simulink model "HalfBridgeCapacitanceModeled"  (R2016a)
settings: Solver=FixedStepDiscrete  StartTime=0.0  StopTime=3e-6  FixedStep=SampleTime  RelTol=1e-3
values from neighbouring files (symbols this model uses):
  Dbot = 49    [HalfBridgeCapacitanceModelling.m]
  DelayBot = 50    [HalfBridgeCapacitanceModelling.m]
  DelayTop = 0    [HalfBridgeCapacitanceModelling.m]
  Dtop = 49    [HalfBridgeCapacitanceModelling.m]
  fsw = 1000e3    (= 1000000)    [HalfBridgeCapacitanceModelling.m]
  Rg = 1.5    [HalfBridgeCapacitanceModelling.m]
  Rload = 200/15    (= 13.3333333333)    [HalfBridgeCapacitanceModelling.m]
  Roff = 5    [HalfBridgeCapacitanceModelling.m]
  Ron = 20    [HalfBridgeCapacitanceModelling.m]
libraries: nesl_utility x32, elec_lib x28, fl_lib x26
(part 1 of 2)
settings Model: SimulationMode=accelerator  Creator=ugurm  LastModifiedBy=kkfrk
settings OptimizationCC: EfficientMapNaN2IntZero=off
settings HardwareCC: TargetBitPerPointer=64  TargetLongLongMode=on  TargetIntDivRoundTo=Zero  TargetEndianess=LittleEndian  TargetWordSize=64  TargetHWDeviceType=MATLAB Host  ProdEqTarget=off
settings CodeAppCC: MaxIdLength=128
settings GRTTargetCC: GeneratePreprocessorConditionals=Use local settings  CombineOutputUpdateFcns=off  GRTInterface=on

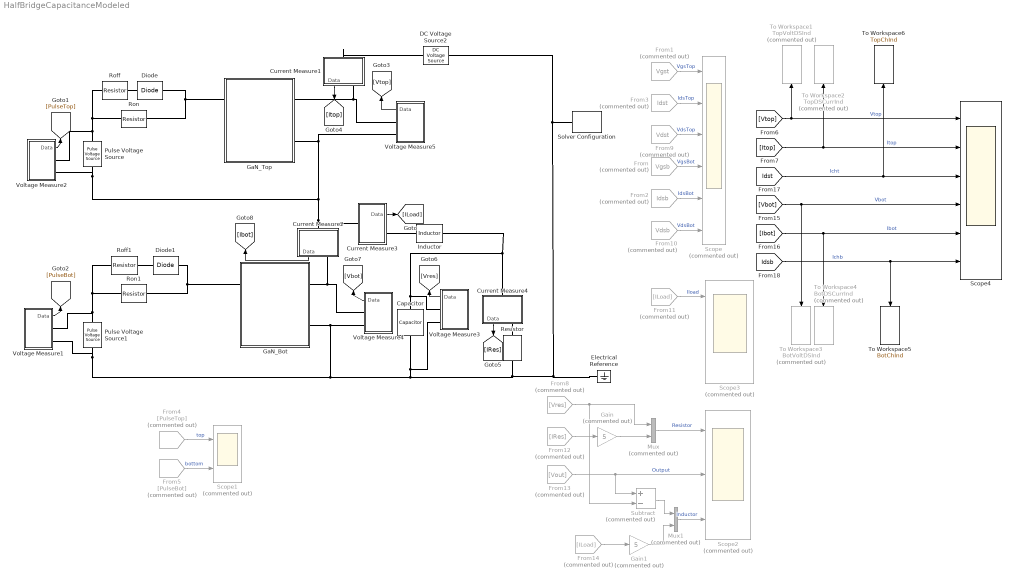
== system HalfBridgeCapacitanceModeled ==
  Capacitor : elec_lib/Passive Devices/Capacitor  enable_table=0  c=Cload F  Cvec=[ 1e-5 1e-6 ] F  Vvec=[ 0 10 ] V  CV_table_symmetry=1  C_tol=5  enable_C_tol=0  tol_distribution=1  nSigma=4  r=1e-6 Ohm  g=0 1/Ohm  initV=0 V  enable_operating_limits=0  operating_limit_action=2  max_working_voltage_range=[ -25 25 ] V  power_rating=1 W  enable_faults=0  fault_action=1  Cscale_faulted=100  R_faulted=0.001 Ohm  G_faulted=0 1/Ohm  tau_fault=0.001 s  enable_temporal_fault=0  t_fault=1 s  enable_behavioral_fault=0  max_permissible_voltage_range=[ -100 100 ] V  t_fail_on_voltage=1 s
  Current Measure1 : Subsystem
  Current Measure2 : Subsystem
  Current Measure3 : Subsystem
  Current Measure4 : Subsystem
  DC Voltage Source2 : elec_lib/Additional Components/SPICE-Compatible Components/Sources/DC Voltage Source  DC=Vdc V
  Diode : elec_lib/Semiconductor Devices/Diode  ModelType=1  Vf=0.6 V  Ron=0.3 Ohm  Goff=1e-8 S  Rz=0.3 Ohm  Vz=50 V  C_PWL=5 pF  prmExp=1  I12=[ 0.0137 0.545 ] A  V12=[ 0.6 0.7 ] V  I1=0.0137 A  V1=0.6 V  RS=0.01 Ohm  IS=1e-12 A  Tmeas=25 degC  ec=1  BV=Inf V  C_param=1  CJ0=5 pF  VJ=1 V  Mgrad=0.5  Vvec=[ 0.1 10 100 ] V  Cvec=[ 3.5 1 0.4 ] pF  FC=0.5  Q_param=1  Irrm=-7.15 A  iF=4 A  didt=-750 A/us  trr=115 ns  TT=50 ns  tau=100 ns  T_param=1  IS_T2=1.25e-7 A  I1_T2=0.245 A  V1_T2=0.5 V  Tmeas2=125 degC  EG_param=1  EG=1.11 eV  XTI_param=1  XTI=3  dBVdT=0 V/K  Tdevice=25 degC  Rth=[ 0 10 ] K/W  thermal_mass_parameterization=1  thermal_mass=[ 0 1 ] J/K  thermal_time_constant=[ 0 10 ] s  thermal_mass_initial_temperatures=[ 25 25 ] degC
  Diode1 : elec_lib/Semiconductor Devices/Diode  ModelType=1  Vf=0.6 V  Ron=0.3 Ohm  Goff=1e-8 S  Rz=0.3 Ohm  Vz=50 V  C_PWL=5 pF  prmExp=1  I12=[ 0.0137 0.545 ] A  V12=[ 0.6 0.7 ] V  I1=0.0137 A  V1=0.6 V  RS=0.01 Ohm  IS=1e-12 A  Tmeas=25 degC  ec=1  BV=Inf V  C_param=1  CJ0=5 pF  VJ=1 V  Mgrad=0.5  Vvec=[ 0.1 10 100 ] V  Cvec=[ 3.5 1 0.4 ] pF  FC=0.5  Q_param=1  Irrm=-7.15 A  iF=4 A  didt=-750 A/us  trr=115 ns  TT=50 ns  tau=100 ns  T_param=1  IS_T2=1.25e-7 A  I1_T2=0.245 A  V1_T2=0.5 V  Tmeas2=125 degC  EG_param=1  EG=1.11 eV  XTI_param=1  XTI=3  dBVdT=0 V/K  Tdevice=25 degC  Rth=[ 0 10 ] K/W  thermal_mass_parameterization=1  thermal_mass=[ 0 1 ] J/K  thermal_time_constant=[ 0 10 ] s  thermal_mass_initial_temperatures=[ 25 25 ] degC
  Electrical Reference : fl_lib/Electrical/Electrical Elements/Electrical Reference
  From : From  Commented=on  GotoTag=Vgsb  TagVisibility=global
  From1 : From  Commented=on  GotoTag=Vgst  TagVisibility=global
  From10 : From  Commented=on  GotoTag=Vdsb  TagVisibility=global
  From11 : From  Commented=on  GotoTag=ILoad
  From12 : From  Commented=on  GotoTag=IRes
  From13 : From  Commented=on  GotoTag=Vout
  From14 : From  Commented=on  GotoTag=ILoad
  From2 : From  Commented=on  GotoTag=Idsb  TagVisibility=global
  From3 : From  Commented=on  GotoTag=Idst  TagVisibility=global
  From4 : From  Commented=on  GotoTag=PulseTop
  From5 : From  Commented=on  GotoTag=PulseBot
  From8 : From  Commented=on  GotoTag=Vres
  From9 : From  Commented=on  GotoTag=Vdst  TagVisibility=global
  GaN_Bot : Subsystem
  GaN_Top : Subsystem
  Gain : Gain  Commented=on  Gain=5
  Gain1 : Gain  Commented=on  Gain=5
  Inductor : elec_lib/Passive Devices/Inductor  l=Lload H  L_tol=20  enable_L_tol=0  tol_distribution=1  nSigma=4  r=0 Ohm  g=1e-9 1/Ohm  initI=0 A  enable_operating_limits=0  operating_limit_action=2  max_working_current=1 A  power_rating=1 W  enable_faults=0  fault_action=1  lambdaPercent=50  k_faulted=0.9999 Ohm  turnsShort=0  openCct=0  groundShort=0  groundShortG=0 1/Ohm  tau_fault=0.001 s  enable_temporal_fault=0  t_fault=1 s  enable_behavioral_fault=0  max_permissible_voltage=100 V  n_fail_on_voltage=1  max_permissible_current=1 A  t_fail_on_current=1 s
  Mux : Mux  Commented=on  Inputs=2
  Mux1 : Mux  Commented=on  Inputs=2
  Pulse Voltage Source : elec_lib/Additional Components/SPICE-Compatible Components/Sources/Pulse Voltage Source  V1=VpulseMin V  V2=VpulseMax V  TD=DelayTop/(100*fsw) s  TR=1e-9 s  TF=1e-9 s  PW=Dtop/(100*fsw) s  PER=1/fsw s
  Pulse Voltage Source1 : elec_lib/Additional Components/SPICE-Compatible Components/Sources/Pulse Voltage Source  V1=VpulseMin V  V2=VpulseMax V  TD=DelayBot/(100*fsw) s  TR=1e-9 s  TF=1e-9 s  PW=Dbot/(100*fsw) s  PER=1/fsw s
  Resistor : elec_lib/Passive Devices/Resistor  R=Rload Ohm  R_tol=5  enable_R_tol=0  tol_distribution=1  nSigma=4  enable_operating_limits=0  operating_limit_action=2  max_working_voltage=100 V  power_rating=1 W  enable_faults=0  fault_action=1  R_faulted=Inf Ohm  enable_temporal_fault=0  t_fault=1 s  enable_behavioral_fault=0  max_permissible_current=1 A  t_fail_on_current=1 s  noise_mode=0  sample_time=0.001 s  repeatability=1  auto_seed=1196140742  user_seed=0  Tdevice=25 degC  alpha=0.00393 1/K  Tmeas=25 degC  thermal_mass=100 J/K  initial_temperature=25 degC  power_derating_T1=70 degC  power_derating_T2=155 degC  operating_temperature_range_vec=[ -50 150 ] degC
  Roff : elec_lib/Passive Devices/Resistor  R=Roff Ohm  R_tol=5  enable_R_tol=0  tol_distribution=1  nSigma=4  enable_operating_limits=0  operating_limit_action=2  max_working_voltage=100 V  power_rating=1 W  enable_faults=0  fault_action=1  R_faulted=Inf Ohm  enable_temporal_fault=0  t_fault=1 s  enable_behavioral_fault=0  max_permissible_current=1 A  t_fail_on_current=1 s  noise_mode=0  sample_time=0.001 s  repeatability=1  auto_seed=2348838240  user_seed=0  Tdevice=25 degC  alpha=0.00393 1/K  Tmeas=25 degC  thermal_mass=100 J/K  initial_temperature=25 degC  power_derating_T1=70 degC  power_derating_T2=155 degC  operating_temperature_range_vec=[ -50 150 ] degC
  Roff1 : elec_lib/Passive Devices/Resistor  R=Roff Ohm  R_tol=5  enable_R_tol=0  tol_distribution=1  nSigma=4  enable_operating_limits=0  operating_limit_action=2  max_working_voltage=100 V  power_rating=1 W  enable_faults=0  fault_action=1  R_faulted=Inf Ohm  enable_temporal_fault=0  t_fault=1 s  enable_behavioral_fault=0  max_permissible_current=1 A  t_fail_on_current=1 s  noise_mode=0  sample_time=0.001 s  repeatability=1  auto_seed=4112460543  user_seed=0  Tdevice=25 degC  alpha=0.00393 1/K  Tmeas=25 degC  thermal_mass=100 J/K  initial_temperature=25 degC  power_derating_T1=70 degC  power_derating_T2=155 degC  operating_temperature_range_vec=[ -50 150 ] degC
  Ron : elec_lib/Passive Devices/Resistor  R=Ron Ohm  R_tol=5  enable_R_tol=0  tol_distribution=1  nSigma=4  enable_operating_limits=0  operating_limit_action=2  max_working_voltage=100 V  power_rating=1 W  enable_faults=0  fault_action=1  R_faulted=Inf Ohm  enable_temporal_fault=0  t_fault=1 s  enable_behavioral_fault=0  max_permissible_current=1 A  t_fail_on_current=1 s  noise_mode=0  sample_time=0.001 s  repeatability=1  auto_seed=4144164703  user_seed=0  Tdevice=25 degC  alpha=0.00393 1/K  Tmeas=25 degC  thermal_mass=100 J/K  initial_temperature=25 degC  power_derating_T1=70 degC  power_derating_T2=155 degC  operating_temperature_range_vec=[ -50 150 ] degC
  Ron1 : elec_lib/Passive Devices/Resistor  R=Ron Ohm  R_tol=5  enable_R_tol=0  tol_distribution=1  nSigma=4  enable_operating_limits=0  operating_limit_action=2  max_working_voltage=100 V  power_rating=1 W  enable_faults=0  fault_action=1  R_faulted=Inf Ohm  enable_temporal_fault=0  t_fault=1 s  enable_behavioral_fault=0  max_permissible_current=1 A  t_fail_on_current=1 s  noise_mode=0  sample_time=0.001 s  repeatability=1  auto_seed=676943032  user_seed=0  Tdevice=25 degC  alpha=0.00393 1/K  Tmeas=25 degC  thermal_mass=100 J/K  initial_temperature=25 degC  power_derating_T1=70 degC  power_derating_T2=155 degC  operating_temperature_range_vec=[ -50 150 ] degC
  Scope : Scope  Commented=on  NumInputPorts=6
  Scope1 : Scope  Commented=on  NumInputPorts=2
  Scope2 : Scope  Commented=on  NumInputPorts=3
  Scope3 : Scope  Commented=on  NumInputPorts=3
  Scope4 : Scope  NumInputPorts=6
  Solver Configuration : nesl_utility/Solver Configuration  PhysicalDomain=network_engine_domain  SubClassName=solver  LeftPortType=input  RightPortType=generic  Accelerate=off  Tones=[]  Harmonics=[]  SimulateNoise=off  Profile=off  UseLocalSampling=off  EnableSwitchedLinearOptims=on  FrequencyDomain=off  UseCCode=off  RelTol=0.001  AbsTol=1e-06  MinStep=1e-09  ToWorkspace=off  RevertToSquareIcSolve=off  NumHomotopyIterations=100  PhasorMode=off  PhasorModeNumHarmonics=1  OverrideAbsTol=off  DoDC=off  ResidualTolerance=1e-09  UseLocalSolver=on  LocalSolverChoice=NE_BACKWARD_EULER_ADVANCER  LocalSolverSampleTime=SampleTime  DoFixedCost=on  MaxNonlinIter=3  MaxModeIter=2  LinearAlgebra=Sparse  DelaysMemoryBudget=1024  AutomaticFiltering=on  FilteringTimeConstant=0.001
  Subtract : Sum  Commented=on  Inputs=+-
  To Workspace1 : ToWorkspace  Commented=on  VariableName=TopVoltDSInd  SampleTime=-1
      settings: Save2DSignal=2-D array (concatenate along first dimension)
  To Workspace2 : ToWorkspace  Commented=on  VariableName=TopDSCurrInd  SampleTime=-1
      settings: Save2DSignal=2-D array (concatenate along first dimension)
  To Workspace3 : ToWorkspace  Commented=on  VariableName=BotVoltDSInd  SampleTime=-1
      settings: Save2DSignal=2-D array (concatenate along first dimension)
  To Workspace4 : ToWorkspace  Commented=on  VariableName=BotDSCurrInd  SampleTime=-1
      settings: Save2DSignal=2-D array (concatenate along first dimension)
  To Workspace5 : ToWorkspace  VariableName=BotChInd  SampleTime=-1
      settings: Save2DSignal=2-D array (concatenate along first dimension)
  To Workspace6 : ToWorkspace  VariableName=TopChInd  SampleTime=-1
      settings: Save2DSignal=2-D array (concatenate along first dimension)
  Voltage Measure1 : Subsystem
  Voltage Measure2 : Subsystem
  Voltage Measure3 : Subsystem
  Voltage Measure4 : Subsystem
  Voltage Measure5 : Subsystem
  wires:
  Current Measure3/1(Data) -> [ILoad]
  From/1 -> Scope/4  "VgsBot"
  From2/1 -> Scope/5  "IdsBot"
  From3/1 -> Scope/2  "IdsTop"
  From1/1 -> Scope/1  "VgsTop"
  From9/1 -> Scope/3  "VdsTop"
  From10/1 -> Scope/6  "VdsBot"
  From11/1 -> Scope3/1  "Iload"
  From4/1 -> Scope1/1  "top"
  From5/1 -> Scope1/2  "bottom"
  Voltage Measure2/1(Data) -> [PulseTop]
  Voltage Measure1/1(Data) -> [PulseBot]
  Current Measure4/1(Data) -> [IRes]
  Voltage Measure3/1(Data) -> [Vres]
  Voltage Measure4/1(Data) -> [Vbot]
  From8/1 -> Mux/1, Subtract/2
  From12/1 -> Gain/1
  Mux/1 -> Scope2/1  "Resistor"
  From13/1 -> Scope2/2, Subtract/1  "Output"
  Mux1/1 -> Scope2/3  "Inductor"
  From14/1 -> Gain1/1
  Subtract/1 -> Mux1/1
  Gain/1 -> Mux/2
  Gain1/1 -> Mux1/2
  Voltage Measure5/1(Data) -> [Vtop]
  Current Measure1/1(Data) -> [Itop]
  Current Measure2/1(Data) -> [Ibot]
  [Vtop] -> To Workspace1/1, Scope4/1  "Vtop"
  [Itop] -> Scope4/2, To Workspace2/1  "Itop"
  [Idsb] -> To Workspace5/1, Scope4/6  "Ichb"
  [Ibot] -> To Workspace4/1, Scope4/5  "Ibot"
  [Vbot] -> To Workspace3/1, Scope4/4  "Vbot"
  [Idst] -> To Workspace6/1, Scope4/3  "Icht"
  connections:
  Ron/RConn1 -- Roff/RConn1 -- Voltage Measure2/RConn1 -- Pulse Voltage Source/LConn1
  Ron/LConn1 -- Diode/LConn1 -- GaN_Top/LConn1
  Current Measure3/LConn1 -- Current Measure2/LConn1 -- Voltage Measure5/RConn2 -- GaN_Top/RConn2 -- Voltage Measure2/RConn2 -- Pulse Voltage Source/RConn1
  Ron1/RConn1 -- Pulse Voltage Source1/LConn1 -- Voltage Measure1/RConn1 -- Roff1/RConn1
  Ron1/LConn1 -- Diode1/LConn1 -- GaN_Bot/LConn1
  Inductor/RConn1 -- Current Measure4/LConn1 -- Capacitor/LConn1 -- Voltage Measure3/RConn1
  Voltage Measure4/RConn2 -- GaN_Bot/RConn2 -- Voltage Measure1/RConn2 -- Pulse Voltage Source1/RConn1 -- Electrical Reference/LConn1 -- DC Voltage Source2/RConn1 -- Solver Configuration/RConn1 -- Resistor/RConn1 -- Capacitor/RConn1 -- Voltage Measure3/RConn2
  Roff/LConn1 -- Diode/RConn1
  Roff1/LConn1 -- Diode1/RConn1
  Current Measure3/RConn1 -- Inductor/LConn1
  Current Measure4/RConn1 -- Resistor/LConn1
  GaN_Top/RConn1 -- Current Measure1/RConn1 -- Voltage Measure5/RConn1
  Current Measure1/LConn1 -- DC Voltage Source2/LConn1
  GaN_Bot/RConn1 -- Current Measure2/RConn1 -- Voltage Measure4/RConn1

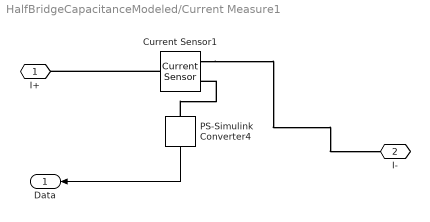
== system HalfBridgeCapacitanceModeled/Current Measure1 ==
  Current Sensor1 : fl_lib/Electrical/Electrical Sensors/Current Sensor
  PS-Simulink Converter4 : nesl_utility/PS-Simulink Converter  PhysicalDomain=network_engine_domain  SubClassName=ps_output  LeftPortType=input  RightPortType=output  PseudoPeriodic=off  Frequencies=[]  Unit=1  AffineConversion=off
  I+ : PMIOPort  Port=1  Side=Left
  I- : PMIOPort  Port=2  Side=Right
  Data : Outport
  wires:
  PS-Simulink Converter4/1 -> Data/1
  connections:
  Current Sensor1/RConn2 -- I-/RConn1
  PS-Simulink Converter4/LConn1 -- Current Sensor1/RConn1
  Current Sensor1/LConn1 -- I+/RConn1

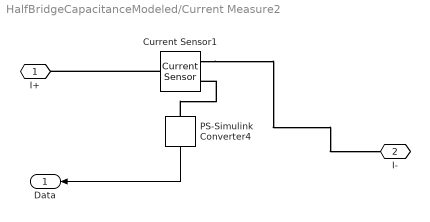
== system HalfBridgeCapacitanceModeled/Current Measure2 ==
  Current Sensor1 : fl_lib/Electrical/Electrical Sensors/Current Sensor
  PS-Simulink Converter4 : nesl_utility/PS-Simulink Converter  PhysicalDomain=network_engine_domain  SubClassName=ps_output  LeftPortType=input  RightPortType=output  PseudoPeriodic=off  Frequencies=[]  Unit=1  AffineConversion=off
  I+ : PMIOPort  Port=1  Side=Left
  I- : PMIOPort  Port=2  Side=Right
  Data : Outport
  wires:
  PS-Simulink Converter4/1 -> Data/1
  connections:
  Current Sensor1/RConn2 -- I-/RConn1
  PS-Simulink Converter4/LConn1 -- Current Sensor1/RConn1
  Current Sensor1/LConn1 -- I+/RConn1

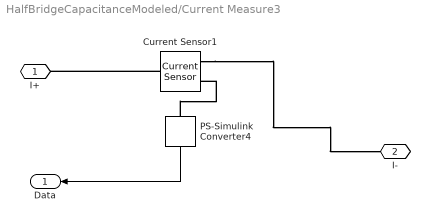
== system HalfBridgeCapacitanceModeled/Current Measure3 ==
  Current Sensor1 : fl_lib/Electrical/Electrical Sensors/Current Sensor
  PS-Simulink Converter4 : nesl_utility/PS-Simulink Converter  PhysicalDomain=network_engine_domain  SubClassName=ps_output  LeftPortType=input  RightPortType=output  PseudoPeriodic=off  Frequencies=[]  Unit=1  AffineConversion=off
  I+ : PMIOPort  Port=1  Side=Left
  I- : PMIOPort  Port=2  Side=Right
  Data : Outport
  wires:
  PS-Simulink Converter4/1 -> Data/1
  connections:
  Current Sensor1/LConn1 -- I+/RConn1
  PS-Simulink Converter4/LConn1 -- Current Sensor1/RConn1
  Current Sensor1/RConn2 -- I-/RConn1

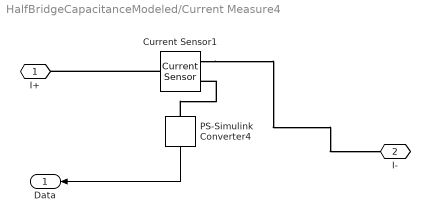
== system HalfBridgeCapacitanceModeled/Current Measure4 ==
  Current Sensor1 : fl_lib/Electrical/Electrical Sensors/Current Sensor
  PS-Simulink Converter4 : nesl_utility/PS-Simulink Converter  PhysicalDomain=network_engine_domain  SubClassName=ps_output  LeftPortType=input  RightPortType=output  PseudoPeriodic=off  Frequencies=[]  Unit=1  AffineConversion=off
  I+ : PMIOPort  Port=1  Side=Left
  I- : PMIOPort  Port=2  Side=Right
  Data : Outport
  wires:
  PS-Simulink Converter4/1 -> Data/1
  connections:
  Current Sensor1/RConn2 -- I-/RConn1
  PS-Simulink Converter4/LConn1 -- Current Sensor1/RConn1
  Current Sensor1/LConn1 -- I+/RConn1

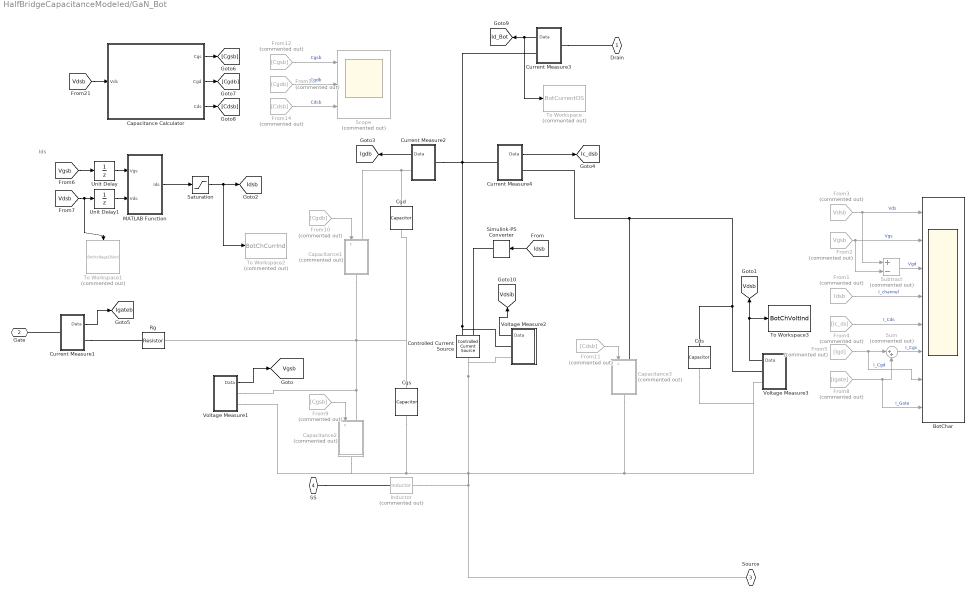
== system HalfBridgeCapacitanceModeled/GaN_Bot ==
  note: Ids
  BotChar : Scope  NumInputPorts=8
  Capacitance Calculator : Subsystem
  Capacitance1 : Subsystem  Commented=on
  Capacitance2 : Subsystem  Commented=on
  Capacitance3 : Subsystem  Commented=on
  Cds : elec_lib/Passive Devices/Capacitor  enable_table=0  c=Cds F  Cvec=[ 1e-5 1e-6 ] F  Vvec=[ 0 10 ] V  CV_table_symmetry=1  C_tol=5  enable_C_tol=0  tol_distribution=1  nSigma=4  r=1e-6 Ohm  g=0 1/Ohm  initV=0 V  enable_operating_limits=0  operating_limit_action=1  max_working_voltage_range=[ -25 25 ] V  power_rating=1 W  enable_faults=0  fault_action=1  Cscale_faulted=100  R_faulted=0.001 Ohm  G_faulted=0 1/Ohm  tau_fault=0.001 s  enable_temporal_fault=0  t_fault=1 s  enable_behavioral_fault=0  max_permissible_voltage_range=[ -100 100 ] V  t_fail_on_voltage=1 s
  Cgd : elec_lib/Passive Devices/Capacitor  enable_table=0  c=Cgd F  Cvec=[ 1e-5 1e-6 ] F  Vvec=[ 0 10 ] V  CV_table_symmetry=1  C_tol=5  enable_C_tol=0  tol_distribution=1  nSigma=4  r=1e-6 Ohm  g=0 1/Ohm  initV=0 V  enable_operating_limits=0  operating_limit_action=2  max_working_voltage_range=[ -25 25 ] V  power_rating=1 W  enable_faults=0  fault_action=1  Cscale_faulted=100  R_faulted=0.001 Ohm  G_faulted=0 1/Ohm  tau_fault=0.001 s  enable_temporal_fault=0  t_fault=1 s  enable_behavioral_fault=0  max_permissible_voltage_range=[ -100 100 ] V  t_fail_on_voltage=1 s
  Cgs : elec_lib/Passive Devices/Capacitor  enable_table=0  c=Cgs F  Cvec=[ 1e-5 1e-6 ] F  Vvec=[ 0 10 ] V  CV_table_symmetry=1  C_tol=5  enable_C_tol=0  tol_distribution=1  nSigma=4  r=1e-6 Ohm  g=0 1/Ohm  initV=0 V  enable_operating_limits=0  operating_limit_action=2  max_working_voltage_range=[ -25 25 ] V  power_rating=1 W  enable_faults=0  fault_action=1  Cscale_faulted=100  R_faulted=0.001 Ohm  G_faulted=0 1/Ohm  tau_fault=0.001 s  enable_temporal_fault=0  t_fault=1 s  enable_behavioral_fault=0  max_permissible_voltage_range=[ -100 100 ] V  t_fail_on_voltage=1 s
  Controlled Current Source : fl_lib/Electrical/Electrical Sources/Controlled Current Source
  Current Measure1 : Subsystem
  Current Measure2 : Subsystem
  Current Measure3 : Subsystem
  Current Measure4 : Subsystem
  From1 : From  Commented=on  GotoTag=Idsb  TagVisibility=global
  From10 : From  Commented=on  GotoTag=Cgdb
  From11 : From  Commented=on  GotoTag=Cdsb
  From12 : From  Commented=on  GotoTag=Cgsb
  From13 : From  Commented=on  GotoTag=Cgdb
  From14 : From  Commented=on  GotoTag=Cdsb
  From2 : From  Commented=on  GotoTag=Vgsb  TagVisibility=global
  From3 : From  Commented=on  GotoTag=Vdsb  TagVisibility=global
  From4 : From  Commented=on  GotoTag=Ic_ds
  From5 : From  Commented=on  GotoTag=Igd
  From8 : From  Commented=on  GotoTag=Igate
  From9 : From  Commented=on  GotoTag=Cgsb
  Inductor : elec_lib/Passive Devices/Inductor  Commented=on  l=Lss H  L_tol=20  enable_L_tol=0  tol_distribution=1  nSigma=4  r=0 Ohm  g=1e-9 1/Ohm  initI=0 A  enable_operating_limits=0  operating_limit_action=1  max_working_current=1 A  power_rating=1 W  enable_faults=0  fault_action=1  lambdaPercent=50  k_faulted=0.9999 Ohm  turnsShort=0  openCct=0  groundShort=0  groundShortG=0 1/Ohm  tau_fault=0.001 s  enable_temporal_fault=0  t_fault=1 s  enable_behavioral_fault=0  max_permissible_voltage=100 V  n_fail_on_voltage=1  max_permissible_current=1 A  t_fail_on_current=1 s
  MATLAB Function : MATLAB Function  TreatAsAtomicUnit=on
  Rg : elec_lib/Passive Devices/Resistor  R=Rg Ohm  R_tol=5  enable_R_tol=0  tol_distribution=1  nSigma=4  enable_operating_limits=0  operating_limit_action=2  max_working_voltage=100 V  power_rating=1 W  enable_faults=0  fault_action=1  R_faulted=Inf Ohm  enable_temporal_fault=0  t_fault=1 s  enable_behavioral_fault=0  max_permissible_current=1 A  t_fail_on_current=1 s  noise_mode=0  sample_time=0.001 s  repeatability=1  auto_seed=3890346746  user_seed=0  Tdevice=25 degC  alpha=0.00393 1/K  Tmeas=25 degC  thermal_mass=100 J/K  initial_temperature=25 degC  power_derating_T1=70 degC  power_derating_T2=155 degC  operating_temperature_range_vec=[ -50 150 ] degC
  Saturation : Saturate  UpperLimit=200  LowerLimit=-200
  Scope : Scope  Commented=on  NumInputPorts=3
  Simulink-PS Converter : nesl_utility/Simulink-PS Converter  PhysicalDomain=network_engine_domain  SubClassName=ps_input  LeftPortType=input  RightPortType=output  PseudoPeriodic=off  Frequencies=[]  NoiseDistribution=none  NoiseParameters=[]  Unit=1  AffineConversion=off  InputFiltering=off  SimscapeFilterOrder=1  InputFilterTimeConstant=0.001  UdotUserProvided=1
  Subtract : Sum  Commented=on  Inputs=+-
  Sum : Sum  Commented=on  Inputs=|++
  To Workspace : ToWorkspace  Commented=on  VariableName=BotCurrentDS  SampleTime=-1
      settings: Save2DSignal=2-D array (concatenate along first dimension)
  To Workspace1 : ToWorkspace  Commented=on  VariableName=BotVoltageDSInd  SampleTime=-1
      settings: Save2DSignal=2-D array (concatenate along first dimension)
  To Workspace2 : ToWorkspace  Commented=on  VariableName=BotChCurrInd  SampleTime=-1
      settings: Save2DSignal=2-D array (concatenate along first dimension)
  To Workspace3 : ToWorkspace  VariableName=BotChVoltInd  SampleTime=-1
      settings: Save2DSignal=2-D array (concatenate along first dimension)
  Unit Delay : UnitDelay  SampleTime=-1
  Unit Delay1 : UnitDelay  SampleTime=-1
  Voltage Measure1 : Subsystem
  Voltage Measure2 : Subsystem
  Voltage Measure3 : Subsystem
  Drain : PMIOPort  Port=1  Side=Right
  Gate : PMIOPort  Port=2  Side=Left
  Source : PMIOPort  Port=3  Side=Right
  SS : PMIOPort  Port=4  Side=Left
  tag scope: Ic_dsb=global, Id_Bot=global, Idsb=global, Igateb=global, Igdb=global, Vdsb=global, Vdsib=global, Vgsb=global
  wires:
  Voltage Measure1/1(Data) -> [Vgsb]
  [Vdsb] -> Unit Delay1/1, To Workspace1/1
  Unit Delay/1 -> MATLAB Function/1(Vgs)
  MATLAB Function/1(Ids) -> Saturation/1
  [Vgsb] -> Unit Delay/1
  [Idsb] -> Simulink-PS Converter/1
  From2/1 -> BotChar/2, Subtract/2  "Vgs"
  From3/1 -> BotChar/1, Subtract/1  "Vds"
  From1/1 -> BotChar/4  "I_channel"
  Subtract/1 -> BotChar/3  "Vgd"
  From4/1 -> BotChar/5  "I_Cds"
  From5/1 -> BotChar/7, Sum/1  "I_Cgd"
  From8/1 -> BotChar/8, Sum/2  "I_Gate"
  Current Measure2/1(Data) -> [Igdb]
  Current Measure4/1(Data) -> [Ic_dsb]
  Sum/1 -> BotChar/6  "I_Cgs"
  Current Measure1/1(Data) -> [Igateb]
  Voltage Measure3/1(Data) -> To Workspace3/1, [Vdsb]
  [Vdsb] -> Capacitance Calculator/1(Vds)
  Capacitance Calculator/1(Cgs) -> [Cgsb]
  Capacitance Calculator/2(Cgd) -> [Cgdb]
  Capacitance Calculator/3(Cds) -> [Cdsb]
  From9/1 -> Capacitance2/1(c)
  From10/1 -> Capacitance1/1(c)
  From11/1 -> Capacitance3/1(c)
  From12/1 -> Scope/1  "Cgsb"
  From13/1 -> Scope/2  "Cgdb"
  From14/1 -> Scope/3  "Cdsb"
  Current Measure3/1(Data) -> To Workspace/1, [Id_Bot]
  Unit Delay1/1 -> MATLAB Function/2(Vds)
  Voltage Measure2/1(Data) -> [Vdsib]
  Saturation/1 -> [Idsb], To Workspace2/1
  connections:
  Simulink-PS Converter/RConn1 -- Controlled Current Source/RConn1
  SS/RConn1 -- Inductor/LConn1
  Current Measure1/LConn1 -- Gate/RConn1
  Voltage Measure3/RConn1 -- Cds/LConn1 -- Capacitance3/LConn1 -- Current Measure4/RConn1
  Current Measure1/RConn1 -- Rg/RConn1
  Capacitance1/LConn1 -- Current Measure2/RConn1 -- Cgd/LConn1
  Current Measure3/LConn1 -- Drain/RConn1
  Controlled Current Source/RConn2 -- Voltage Measure2/RConn1 -- Current Measure3/RConn1 -- Current Measure2/LConn1 -- Current Measure4/LConn1
  Inductor/RConn1 -- Source/RConn1 -- Voltage Measure2/RConn2 -- Controlled Current Source/LConn1 -- Voltage Measure1/RConn2 -- Capacitance2/RConn1 -- Cgs/RConn1 -- Cds/RConn1 -- Voltage Measure3/RConn2 -- Capacitance3/RConn1
  Capacitance2/LConn1 -- Voltage Measure1/RConn1 -- Rg/LConn1 -- Cgd/RConn1 -- Cgs/LConn1 -- Capacitance1/RConn1

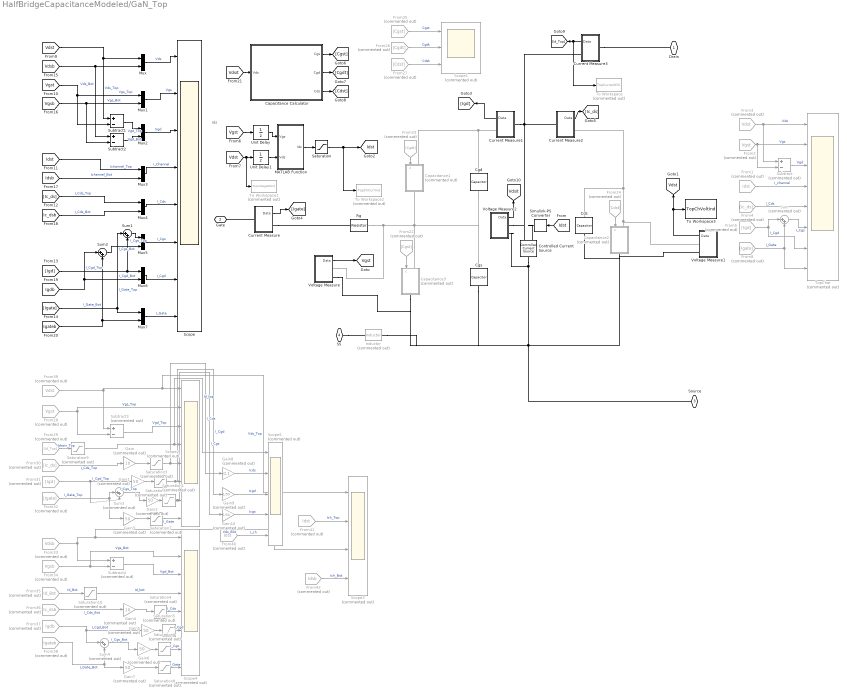
== system HalfBridgeCapacitanceModeled/GaN_Top ==
  note: Ids
  Capacitance Calculator : Subsystem
  Capacitance1 : Subsystem  Commented=on
  Capacitance2 : Subsystem  Commented=on
  Capacitance3 : Subsystem  Commented=on
  Cds : elec_lib/Passive Devices/Capacitor  enable_table=0  c=Cds F  Cvec=[ 1e-5 1e-6 ] F  Vvec=[ 0 10 ] V  CV_table_symmetry=1  C_tol=5  enable_C_tol=0  tol_distribution=1  nSigma=4  r=1e-6 Ohm  g=0 1/Ohm  initV=0 V  enable_operating_limits=0  operating_limit_action=1  max_working_voltage_range=[ -25 25 ] V  power_rating=1 W  enable_faults=0  fault_action=1  Cscale_faulted=100  R_faulted=0.001 Ohm  G_faulted=0 1/Ohm  tau_fault=0.001 s  enable_temporal_fault=0  t_fault=1 s  enable_behavioral_fault=0  max_permissible_voltage_range=[ -100 100 ] V  t_fail_on_voltage=1 s
  Cgd : elec_lib/Passive Devices/Capacitor  enable_table=0  c=Cgd F  Cvec=[ 1e-5 1e-6 ] F  Vvec=[ 0 10 ] V  CV_table_symmetry=1  C_tol=5  enable_C_tol=0  tol_distribution=1  nSigma=4  r=1e-6 Ohm  g=0 1/Ohm  initV=0 V  enable_operating_limits=0  operating_limit_action=1  max_working_voltage_range=[ -25 25 ] V  power_rating=1 W  enable_faults=0  fault_action=1  Cscale_faulted=100  R_faulted=0.001 Ohm  G_faulted=0 1/Ohm  tau_fault=0.001 s  enable_temporal_fault=0  t_fault=1 s  enable_behavioral_fault=0  max_permissible_voltage_range=[ -100 100 ] V  t_fail_on_voltage=1 s
  Cgs : elec_lib/Passive Devices/Capacitor  enable_table=0  c=Cgs F  Cvec=[ 1e-5 1e-6 ] F  Vvec=[ 0 10 ] V  CV_table_symmetry=1  C_tol=5  enable_C_tol=0  tol_distribution=1  nSigma=4  r=1e-6 Ohm  g=0 1/Ohm  initV=0 V  enable_operating_limits=0  operating_limit_action=2  max_working_voltage_range=[ -25 25 ] V  power_rating=1 W  enable_faults=0  fault_action=1  Cscale_faulted=100  R_faulted=0.001 Ohm  G_faulted=0 1/Ohm  tau_fault=0.001 s  enable_temporal_fault=0  t_fault=1 s  enable_behavioral_fault=0  max_permissible_voltage_range=[ -100 100 ] V  t_fail_on_voltage=1 s
  Controlled Current Source : fl_lib/Electrical/Electrical Sources/Controlled Current Source
  Current Measure : Subsystem
  Current Measure1 : Subsystem
  Current Measure2 : Subsystem
  Current Measure3 : Subsystem
  From1 : From  Commented=on  GotoTag=Idst  TagVisibility=global
  From2 : From  Commented=on  GotoTag=Vgst  TagVisibility=global
  From22 : From  Commented=on  GotoTag=Cgst
  From23 : From  Commented=on  GotoTag=Cgdt
  From24 : From  Commented=on  GotoTag=Cdst
  From25 : From  Commented=on  GotoTag=Cgst
  From26 : From  Commented=on  GotoTag=Cgdt
  From27 : From  Commented=on  GotoTag=Cdst
  From28 : From  Commented=on  GotoTag=Vgst  TagVisibility=global
  From29 : From  Commented=on  GotoTag=Id_Top
  From3 : From  Commented=on  GotoTag=Vdst  TagVisibility=global
  From30 : From  Commented=on  GotoTag=Ic_ds
  From31 : From  Commented=on  GotoTag=Igd
  From32 : From  Commented=on  GotoTag=Igate
  From33 : From  Commented=on  GotoTag=Vdsb  TagVisibility=global
  From34 : From  Commented=on  GotoTag=Vgsb  TagVisibility=global
  From35 : From  Commented=on  GotoTag=Id_Bot  TagVisibility=global
  From36 : From  Commented=on  GotoTag=Ic_dsb  TagVisibility=global
  From37 : From  Commented=on  GotoTag=Igdb  TagVisibility=global
  From38 : From  Commented=on  GotoTag=Igateb  TagVisibility=global
  From39 : From  Commented=on  GotoTag=Vdst  TagVisibility=global
  From4 : From  Commented=on  GotoTag=Ic_ds
  From40 : From  Commented=on  GotoTag=Idst  TagVisibility=global
  From41 : From  Commented=on  GotoTag=Idst  TagVisibility=global
  From42 : From  Commented=on  GotoTag=Idsb  TagVisibility=global
  From5 : From  Commented=on  GotoTag=Igd
  From8 : From  Commented=on  GotoTag=Igate
  Gain : Gain  Commented=on  Gain=10
  Gain{1..3,5..7} (6 alike) : Gain  Commented=on  Gain=50
  Gain10 : Gain  Commented=on  Gain=1/50
  Gain4 : Gain  Commented=on  Gain=10
  Gain8 : Gain  Commented=on  Gain=0.1
  Gain9 : Gain  Commented=on  Gain=1/50
  Inductor : elec_lib/Passive Devices/Inductor  Commented=on  l=Lss H  L_tol=20  enable_L_tol=0  tol_distribution=1  nSigma=4  r=0 Ohm  g=1e-9 1/Ohm  initI=0 A  enable_operating_limits=0  operating_limit_action=1  max_working_current=1 A  power_rating=1 W  enable_faults=0  fault_action=1  lambdaPercent=50  k_faulted=0.9999 Ohm  turnsShort=0  openCct=0  groundShort=0  groundShortG=0 1/Ohm  tau_fault=0.001 s  enable_temporal_fault=0  t_fault=1 s  enable_behavioral_fault=0  max_permissible_voltage=100 V  n_fail_on_voltage=1  max_permissible_current=1 A  t_fail_on_current=1 s
  MATLAB Function : MATLAB Function  TreatAsAtomicUnit=on
  Mux{,1..7} (8 alike) : Mux  Inputs=2
  Rg : elec_lib/Passive Devices/Resistor  R=Rg Ohm  R_tol=5  enable_R_tol=0  tol_distribution=1  nSigma=4  enable_operating_limits=0  operating_limit_action=2  max_working_voltage=100 V  power_rating=1 W  enable_faults=0  fault_action=1  R_faulted=Inf Ohm  enable_temporal_fault=0  t_fault=1 s  enable_behavioral_fault=0  max_permissible_current=1 A  t_fail_on_current=1 s  noise_mode=0  sample_time=0.001 s  repeatability=1  auto_seed=2715962282  user_seed=0  Tdevice=25 degC  alpha=0.00393 1/K  Tmeas=25 degC  thermal_mass=100 J/K  initial_temperature=25 degC  power_derating_T1=70 degC  power_derating_T2=155 degC  operating_temperature_range_vec=[ -50 150 ] degC
  Saturation : Saturate  UpperLimit=200  LowerLimit=-200
  Saturation{1..2,5..10} (8 alike) : Saturate  Commented=on  UpperLimit=100  LowerLimit=-100
  Saturation3 : Saturate  Commented=on  UpperLimit=250  LowerLimit=-100
  Saturation4 : Saturate  Commented=on  UpperLimit=250  LowerLimit=-100
  Scope : Scope  NumInputPorts=8
  Scope1 : Scope  Commented=on  NumInputPorts=3
  Scope2 : Scope  Commented=on  NumInputPorts=8
  Scope3 : Scope  Commented=on  NumInputPorts=4
  Scope4 : Scope  Commented=on  NumInputPorts=8
  Scope5 : Scope  Commented=on  NumInputPorts=5
  Simulink-PS Converter : nesl_utility/Simulink-PS Converter  PhysicalDomain=network_engine_domain  SubClassName=ps_input  LeftPortType=input  RightPortType=output  PseudoPeriodic=off  Frequencies=[]  NoiseDistribution=none  NoiseParameters=[]  Unit=1  AffineConversion=off  InputFiltering=off  SimscapeFilterOrder=1  InputFilterTimeConstant=0.001  UdotUserProvided=1
  Subtract : Sum  Commented=on  Inputs=+-
  Subtract1 : Sum  Inputs=+-
  Subtract2 : Sum  Inputs=+-
  Subtract3 : Sum  Commented=on  Inputs=+-
  Subtract4 : Sum  Commented=on  Inputs=+-
  Sum : Sum  Commented=on  Inputs=|++
  Sum1 : Sum  Inputs=|++
  Sum2 : Sum  Inputs=|++
  Sum3 : Sum  Commented=on  Inputs=|++
  Sum4 : Sum  Commented=on  Inputs=|++
  To Workspace : ToWorkspace  Commented=on  VariableName=TopCurrentDS  SampleTime=-1
      settings: Save2DSignal=2-D array (concatenate along first dimension)
  To Workspace1 : ToWorkspace  Commented=on  VariableName=TopVoltageDSInd  SampleTime=-1
      settings: Save2DSignal=2-D array (concatenate along first dimension)
  To Workspace2 : ToWorkspace  Commented=on  VariableName=TopChCurrInd  SampleTime=-1
      settings: Save2DSignal=2-D array (concatenate along first dimension)
  To Workspace3 : ToWorkspace  VariableName=TopChVoltInd  SampleTime=-1
      settings: Save2DSignal=2-D array (concatenate along first dimension)
  TopChar : Scope  Commented=on  NumInputPorts=8
  Unit Delay : UnitDelay  SampleTime=-1
  Unit Delay1 : UnitDelay  SampleTime=-1
  Voltage Measure : Subsystem
  Voltage Measure1 : Subsystem
  Voltage Measure2 : Subsystem
  Drain : PMIOPort  Port=1  Side=Right
  Gate : PMIOPort  Port=2  Side=Left
  Source : PMIOPort  Port=3  Side=Right
  SS : PMIOPort  Port=4  Side=Left
  tag scope: Idst=global, Vdsit=global, Vdst=global, Vgst=global
  wires:
  [Vgst] -> Unit Delay/1
  MATLAB Function/1(Ids) -> Saturation/1
  Unit Delay/1 -> MATLAB Function/1(Vgs)
  [Idst] -> Simulink-PS Converter/1
  From2/1 -> Subtract/2, TopChar/2  "Vgs"
  From3/1 -> Subtract/1, TopChar/1  "Vds"
  From1/1 -> TopChar/4  "I_channel"
  Subtract/1 -> TopChar/3  "Vgd"
  Current Measure1/1(Data) -> [Igd]
  Current Measure2/1(Data) -> [Ic_ds]
  From5/1 -> TopChar/7, Sum/1  "I_Cgd"
  From8/1 -> TopChar/8, Sum/2  "I_Gate"
  From4/1 -> TopChar/5  "I_Cds"
  Sum/1 -> TopChar/6  "I_Cgs"
  Current Measure/1(Data) -> [Igate]
  Voltage Measure/1(Data) -> [Vgst]
  [Vdst] -> Mux/1, Subtract1/1  "Vds_Top"
  [Vgst] -> Mux1/1, Subtract1/2  "Vgs_Top"
  [Ic_ds] -> Mux4/1  "I_Cds_Top"
  [Igd] -> Mux6/1, Sum1/2  "I_Cgd_Top"
  [Igate] -> Mux7/1, Sum1/1  "I_Gate_Top"
  Sum1/1 -> Mux5/1  "I_Cgs_Top"
  [Vdsb] -> Subtract2/1, Mux/2  "Vds_Bot"
  [Vgsb] -> Mux1/2, Subtract2/2  "Vgs_Bot"
  [Ic_dsb] -> Mux4/2  "I_Cds_Bot"
  [Igdb] -> Mux6/2, Sum2/1  "I_Cgd_Bot"
  [Igateb] -> Mux7/2, Sum2/2  "I_Gate_Bot"
  Sum2/1 -> Mux5/2  "I_Cgs_Bot"
  Subtract1/1 -> Mux2/1  "Vgd_Top"
  Subtract2/1 -> Mux2/2  "Vgd_Bot"
  [Idst] -> Mux3/1  "Ichannel_Top"
  [Idsb] -> Mux3/2  "Ichannel_Bot"
  Mux7/1 -> Scope/8  "I_Gate"
  Mux6/1 -> Scope/7  "I_Cgd"
  Mux5/1 -> Scope/6  "I_Cgs"
  Mux4/1 -> Scope/5  "I_Cds"
  Mux3/1 -> Scope/4  "I_Channel"
  Mux2/1 -> Scope/3  "Vgd"
  Mux1/1 -> Scope/2  "Vgs"
  Mux/1 -> Scope/1  "Vds"
  [Vdsit] -> Capacitance Calculator/1(Vds)
  Capacitance Calculator/1(Cgs) -> [Cgst]
  Capacitance Calculator/2(Cgd) -> [Cgdt]
  Capacitance Calculator/3(Cds) -> [Cdst]
  From22/1 -> Capacitance3/1(c)
  From23/1 -> Capacitance1/1(c)
  From24/1 -> Capacitance2/1(c)
  From25/1 -> Scope1/1  "Cgst"
  From26/1 -> Scope1/2  "Cgdt"
  From27/1 -> Scope1/3  "Cdst"
  From39/1 -> Scope3/1, Scope2/1, Subtract3/1  "Vds_Top"
  From28/1 -> Scope2/2, Subtract3/2  "Vgs_Top"
  From30/1 -> Gain/1  "I_Cds_Top"
  From31/1 -> Sum3/2, Gain1/1  "I_Cgd_Top"
  From32/1 -> Gain3/1, Sum3/1  "I_Gate_Top"
  From33/1 -> Scope4/1, Scope3/3, Subtract4/1  "Vds_Bot"
  From34/1 -> Scope4/2, Subtract4/2  "Vgs_Bot"
  From36/1 -> Gain4/1  "I_Cds_Bot"
  From37/1 -> Sum4/1, Gain5/1  "I_Cgd_Bot"
  From38/1 -> Gain7/1, Sum4/2  "I_Gate_Bot"
  Subtract3/1 -> Scope2/3  "Vgd_Top"
  Subtract4/1 -> Scope4/3  "Vgd_Bot"
  From29/1 -> Saturation9/1  "Idrain_Top"
  From35/1 -> Saturation10/1  "Id_Bot"
  Sum4/1 -> Gain6/1  "I_Cgs_Bot"
  Gain/1 -> Saturation3/1
  Gain1/1 -> Saturation2/1
  Sum3/1 -> Gain2/1  "I_Cgs_Top"
  Gain3/1 -> Saturation7/1
  Gain4/1 -> Saturation4/1
  Gain6/1 -> Saturation6/1
  Gain7/1 -> Saturation8/1
  Gain2/1 -> Saturation1/1
  Saturation1/1 -> Gain10/1, Scope2/7  "I_Cgs"
  Saturation2/1 -> Gain9/1, Scope2/6  "I_Cgd"
  Saturation3/1 -> Gain8/1, Scope2/5  "I_Cds"
  Saturation4/1 -> Scope4/5  "I_Cds"
  Saturation5/1 -> Scope4/6  "I_Cgd"
  Gain5/1 -> Saturation5/1
  Saturation6/1 -> Scope4/7  "I_Cgs"
  Saturation7/1 -> Scope2/8  "I_Gate"
  Saturation8/1 -> Scope4/8  "I_Gate"
  Current Measure3/1(Data) -> To Workspace/1, [Id_Top]
  Saturation9/1 -> Scope5/1, Scope2/4  "Id_top"
  Saturation10/1 -> Scope4/4  "Id_bot"
  Gain8/1 -> Scope5/2  "Icds"
  Gain9/1 -> Scope5/3  "Icgd"
  Gain10/1 -> Scope5/4  "Icgs"
  From40/1 -> Scope5/5  "I_ch"
  From41/1 -> Scope3/2  "Ich_Top"
  From42/1 -> Scope3/4  "Ich_Bot"
  [Vdst] -> Unit Delay1/1, To Workspace1/1
  Unit Delay1/1 -> MATLAB Function/2(Vds)
  Voltage Measure2/1(Data) -> [Vdsit]
  Saturation/1 -> [Idst], To Workspace2/1
  Voltage Measure1/1(Data) -> To Workspace3/1, [Vdst]
  connections:
  Capacitance1/RConn1 -- Cgs/LConn1 -- Cgd/RConn1 -- Capacitance3/LConn1 -- Rg/LConn1 -- Voltage Measure/RConn1
  Simulink-PS Converter/RConn1 -- Controlled Current Source/RConn1
  SS/RConn1 -- Inductor/LConn1
  Current Measure/LConn1 -- Gate/RConn1
  Capacitance1/LConn1 -- Current Measure1/RConn1 -- Cgd/LConn1
  Capacitance2/LConn1 -- Voltage Measure1/RConn1 -- Cds/LConn1 -- Current Measure2/RConn1
  Current Measure3/LConn1 -- Drain/RConn1
  Controlled Current Source/LConn1 -- Source/RConn1 -- Inductor/RConn1 -- Cgs/RConn1 -- Voltage Measure/RConn2 -- Capacitance3/RConn1 -- Cds/RConn1 -- Voltage Measure1/RConn2 -- Capacitance2/RConn1 -- Voltage Measure2/RConn2
  Current Measure2/LConn1 -- Current Measure3/RConn1 -- Voltage Measure2/RConn1 -- Controlled Current Source/RConn2 -- Current Measure1/LConn1
  Current Measure/RConn1 -- Rg/RConn1

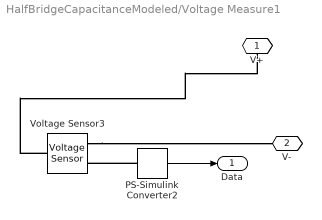
== system HalfBridgeCapacitanceModeled/Voltage Measure1 ==
  PS-Simulink Converter2 : nesl_utility/PS-Simulink Converter  PhysicalDomain=network_engine_domain  SubClassName=ps_output  LeftPortType=input  RightPortType=output  PseudoPeriodic=off  Frequencies=[]  Unit=1  AffineConversion=off
  Voltage Sensor3 : fl_lib/Electrical/Electrical Sensors/Voltage Sensor
  V+ : PMIOPort  Port=1  Side=Right
  V- : PMIOPort  Port=2  Side=Right
  Data : Outport
  wires:
  PS-Simulink Converter2/1 -> Data/1
  connections:
  PS-Simulink Converter2/LConn1 -- Voltage Sensor3/RConn1
  Voltage Sensor3/RConn2 -- V-/RConn1
  Voltage Sensor3/LConn1 -- V+/RConn1

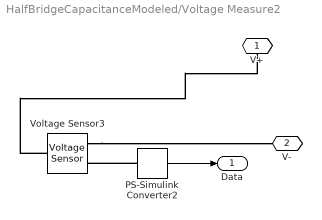
== system HalfBridgeCapacitanceModeled/Voltage Measure2 ==
  PS-Simulink Converter2 : nesl_utility/PS-Simulink Converter  PhysicalDomain=network_engine_domain  SubClassName=ps_output  LeftPortType=input  RightPortType=output  PseudoPeriodic=off  Frequencies=[]  Unit=1  AffineConversion=off
  Voltage Sensor3 : fl_lib/Electrical/Electrical Sensors/Voltage Sensor
  V+ : PMIOPort  Port=1  Side=Right
  V- : PMIOPort  Port=2  Side=Right
  Data : Outport
  wires:
  PS-Simulink Converter2/1 -> Data/1
  connections:
  Voltage Sensor3/LConn1 -- V+/RConn1
  Voltage Sensor3/RConn2 -- V-/RConn1
  PS-Simulink Converter2/LConn1 -- Voltage Sensor3/RConn1

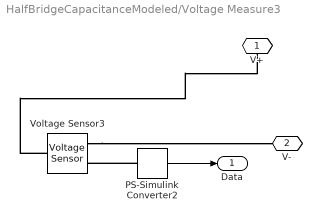
== system HalfBridgeCapacitanceModeled/Voltage Measure3 ==
  PS-Simulink Converter2 : nesl_utility/PS-Simulink Converter  PhysicalDomain=network_engine_domain  SubClassName=ps_output  LeftPortType=input  RightPortType=output  PseudoPeriodic=off  Frequencies=[]  Unit=1  AffineConversion=off
  Voltage Sensor3 : fl_lib/Electrical/Electrical Sensors/Voltage Sensor
  V+ : PMIOPort  Port=1  Side=Right
  V- : PMIOPort  Port=2  Side=Right
  Data : Outport
  wires:
  PS-Simulink Converter2/1 -> Data/1
  connections:
  PS-Simulink Converter2/LConn1 -- Voltage Sensor3/RConn1
  Voltage Sensor3/RConn2 -- V-/RConn1
  Voltage Sensor3/LConn1 -- V+/RConn1

== system HalfBridgeCapacitanceModeled/Voltage Measure4 ==
  PS-Simulink Converter2 : nesl_utility/PS-Simulink Converter  PhysicalDomain=network_engine_domain  SubClassName=ps_output  LeftPortType=input  RightPortType=output  PseudoPeriodic=off  Frequencies=[]  Unit=1  AffineConversion=off
  Voltage Sensor3 : fl_lib/Electrical/Electrical Sensors/Voltage Sensor
  V+ : PMIOPort  Port=1  Side=Right
  V- : PMIOPort  Port=2  Side=Right
  Data : Outport
  wires:
  PS-Simulink Converter2/1 -> Data/1
  connections:
  Voltage Sensor3/LConn1 -- V+/RConn1
  Voltage Sensor3/RConn2 -- V-/RConn1
  PS-Simulink Converter2/LConn1 -- Voltage Sensor3/RConn1

== system HalfBridgeCapacitanceModeled/Voltage Measure5 ==
  PS-Simulink Converter2 : nesl_utility/PS-Simulink Converter  PhysicalDomain=network_engine_domain  SubClassName=ps_output  LeftPortType=input  RightPortType=output  PseudoPeriodic=off  Frequencies=[]  Unit=1  AffineConversion=off
  Voltage Sensor3 : fl_lib/Electrical/Electrical Sensors/Voltage Sensor
  V+ : PMIOPort  Port=1  Side=Right
  V- : PMIOPort  Port=2  Side=Right
  Data : Outport
  wires:
  PS-Simulink Converter2/1 -> Data/1
  connections:
  PS-Simulink Converter2/LConn1 -- Voltage Sensor3/RConn1
  Voltage Sensor3/RConn2 -- V-/RConn1
  Voltage Sensor3/LConn1 -- V+/RConn1

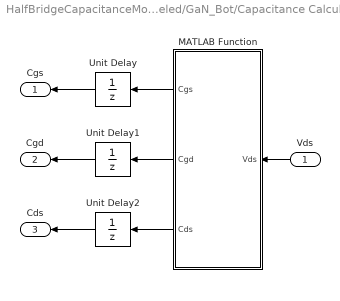
== system HalfBridgeCapacitanceModeled/GaN_Bot/Capacitance Calculator ==
  Vds : Inport
  MATLAB Function : MATLAB Function  TreatAsAtomicUnit=on
  Unit Delay : UnitDelay  InitialCondition=258e-12  SampleTime=-1
  Unit Delay1 : UnitDelay  InitialCondition=63e-12  SampleTime=-1
  Unit Delay2 : UnitDelay  InitialCondition=2e-12  SampleTime=-1
  Cgs : Outport
  Cgd : Outport  Port=2
  Cds : Outport  Port=3
  wires:
  Vds/1 -> MATLAB Function/1(Vds)
  MATLAB Function/1(Cgs) -> Unit Delay/1
  MATLAB Function/2(Cgd) -> Unit Delay1/1
  MATLAB Function/3(Cds) -> Unit Delay2/1
  Unit Delay/1 -> Cgs/1
  Unit Delay1/1 -> Cgd/1
  Unit Delay2/1 -> Cds/1

== system HalfBridgeCapacitanceModeled/GaN_Bot/Capacitance1 ==
  c : Inport
  Simulink-PS Converter : nesl_utility/Simulink-PS Converter  PhysicalDomain=network_engine_domain  SubClassName=ps_input  LeftPortType=input  RightPortType=output  PseudoPeriodic=off  Frequencies=[]  NoiseDistribution=none  NoiseParameters=[]  Unit=1  AffineConversion=off  InputFiltering=off  SimscapeFilterOrder=1  InputFilterTimeConstant=0.001  UdotUserProvided=1
  Variable Capacitor : elec_lib/Passive Devices/Variable Capacitor  prm=2  Cmin=1e-13 F  r=1e-6 Ohm  v0=0 V  q0=0 c
  C+ : PMIOPort  Port=1  Side=Left
  C- : PMIOPort  Port=2  Side=Right
  wires:
  c/1 -> Simulink-PS Converter/1
  connections:
  Variable Capacitor/LConn1 -- Simulink-PS Converter/RConn1
  Variable Capacitor/LConn2 -- C+/RConn1
  Variable Capacitor/RConn1 -- C-/RConn1

== system HalfBridgeCapacitanceModeled/GaN_Bot/Capacitance2 ==
  c : Inport
  Simulink-PS Converter : nesl_utility/Simulink-PS Converter  PhysicalDomain=network_engine_domain  SubClassName=ps_input  LeftPortType=input  RightPortType=output  PseudoPeriodic=off  Frequencies=[]  NoiseDistribution=none  NoiseParameters=[]  Unit=1  AffineConversion=off  InputFiltering=off  SimscapeFilterOrder=1  InputFilterTimeConstant=0.001  UdotUserProvided=1
  Variable Capacitor : elec_lib/Passive Devices/Variable Capacitor  prm=2  Cmin=1e-13 F  r=1e-6 Ohm  v0=0 V  q0=0 c
  C+ : PMIOPort  Port=1  Side=Left
  C- : PMIOPort  Port=2  Side=Right
  wires:
  c/1 -> Simulink-PS Converter/1
  connections:
  Variable Capacitor/RConn1 -- C-/RConn1
  Variable Capacitor/LConn2 -- C+/RConn1
  Variable Capacitor/LConn1 -- Simulink-PS Converter/RConn1

== system HalfBridgeCapacitanceModeled/GaN_Bot/Capacitance3 ==
  c : Inport
  Simulink-PS Converter : nesl_utility/Simulink-PS Converter  PhysicalDomain=network_engine_domain  SubClassName=ps_input  LeftPortType=input  RightPortType=output  PseudoPeriodic=off  Frequencies=[]  NoiseDistribution=none  NoiseParameters=[]  Unit=1  AffineConversion=off  InputFiltering=off  SimscapeFilterOrder=1  InputFilterTimeConstant=0.001  UdotUserProvided=1
  Variable Capacitor : elec_lib/Passive Devices/Variable Capacitor  prm=2  Cmin=1e-13 F  r=1e-6 Ohm  v0=0 V  q0=0 c
  C+ : PMIOPort  Port=1  Side=Left
  C- : PMIOPort  Port=2  Side=Right
  wires:
  c/1 -> Simulink-PS Converter/1
  connections:
  Variable Capacitor/RConn1 -- C-/RConn1
  Variable Capacitor/LConn2 -- C+/RConn1
  Variable Capacitor/LConn1 -- Simulink-PS Converter/RConn1

== system HalfBridgeCapacitanceModeled/GaN_Bot/Current Measure1 ==
  Current Sensor1 : fl_lib/Electrical/Electrical Sensors/Current Sensor
  PS-Simulink Converter4 : nesl_utility/PS-Simulink Converter  PhysicalDomain=network_engine_domain  SubClassName=ps_output  LeftPortType=input  RightPortType=output  PseudoPeriodic=off  Frequencies=[]  Unit=1  AffineConversion=off
  I+ : PMIOPort  Port=1  Side=Left
  I- : PMIOPort  Port=2  Side=Right
  Data : Outport
  wires:
  PS-Simulink Converter4/1 -> Data/1
  connections:
  Current Sensor1/RConn2 -- I-/RConn1
  PS-Simulink Converter4/LConn1 -- Current Sensor1/RConn1
  Current Sensor1/LConn1 -- I+/RConn1

== system HalfBridgeCapacitanceModeled/GaN_Bot/Current Measure2 ==
  Current Sensor1 : fl_lib/Electrical/Electrical Sensors/Current Sensor
  PS-Simulink Converter4 : nesl_utility/PS-Simulink Converter  PhysicalDomain=network_engine_domain  SubClassName=ps_output  LeftPortType=input  RightPortType=output  PseudoPeriodic=off  Frequencies=[]  Unit=1  AffineConversion=off
  I+ : PMIOPort  Port=1  Side=Left
  I- : PMIOPort  Port=2  Side=Right
  Data : Outport
  wires:
  PS-Simulink Converter4/1 -> Data/1
  connections:
  Current Sensor1/RConn2 -- I-/RConn1
  PS-Simulink Converter4/LConn1 -- Current Sensor1/RConn1
  Current Sensor1/LConn1 -- I+/RConn1

== system HalfBridgeCapacitanceModeled/GaN_Bot/Current Measure3 ==
  Current Sensor1 : fl_lib/Electrical/Electrical Sensors/Current Sensor
  PS-Simulink Converter4 : nesl_utility/PS-Simulink Converter  PhysicalDomain=network_engine_domain  SubClassName=ps_output  LeftPortType=input  RightPortType=output  PseudoPeriodic=off  Frequencies=[]  Unit=1  AffineConversion=off
  I+ : PMIOPort  Port=1  Side=Left
  I- : PMIOPort  Port=2  Side=Right
  Data : Outport
  wires:
  PS-Simulink Converter4/1 -> Data/1
  connections:
  Current Sensor1/LConn1 -- I+/RConn1
  PS-Simulink Converter4/LConn1 -- Current Sensor1/RConn1
  Current Sensor1/RConn2 -- I-/RConn1

== system HalfBridgeCapacitanceModeled/GaN_Bot/Current Measure4 ==
  Current Sensor1 : fl_lib/Electrical/Electrical Sensors/Current Sensor
  PS-Simulink Converter4 : nesl_utility/PS-Simulink Converter  PhysicalDomain=network_engine_domain  SubClassName=ps_output  LeftPortType=input  RightPortType=output  PseudoPeriodic=off  Frequencies=[]  Unit=1  AffineConversion=off
  I+ : PMIOPort  Port=1  Side=Left
  I- : PMIOPort  Port=2  Side=Right
  Data : Outport
  wires:
  PS-Simulink Converter4/1 -> Data/1
  connections:
  Current Sensor1/RConn2 -- I-/RConn1
  PS-Simulink Converter4/LConn1 -- Current Sensor1/RConn1
  Current Sensor1/LConn1 -- I+/RConn1

== system HalfBridgeCapacitanceModeled/GaN_Bot/Voltage Measure1 ==
  PS-Simulink Converter2 : nesl_utility/PS-Simulink Converter  PhysicalDomain=network_engine_domain  SubClassName=ps_output  LeftPortType=input  RightPortType=output  PseudoPeriodic=off  Frequencies=[]  Unit=1  AffineConversion=off
  Voltage Sensor3 : fl_lib/Electrical/Electrical Sensors/Voltage Sensor
  V+ : PMIOPort  Port=1  Side=Right
  V- : PMIOPort  Port=2  Side=Right
  Data : Outport
  wires:
  PS-Simulink Converter2/1 -> Data/1
  connections:
  PS-Simulink Converter2/LConn1 -- Voltage Sensor3/RConn1
  Voltage Sensor3/RConn2 -- V-/RConn1
  Voltage Sensor3/LConn1 -- V+/RConn1

== system HalfBridgeCapacitanceModeled/GaN_Bot/Voltage Measure2 ==
  PS-Simulink Converter2 : nesl_utility/PS-Simulink Converter  PhysicalDomain=network_engine_domain  SubClassName=ps_output  LeftPortType=input  RightPortType=output  PseudoPeriodic=off  Frequencies=[]  Unit=1  AffineConversion=off
  Voltage Sensor3 : fl_lib/Electrical/Electrical Sensors/Voltage Sensor
  V+ : PMIOPort  Port=1  Side=Right
  V- : PMIOPort  Port=2  Side=Right
  Data : Outport
  wires:
  PS-Simulink Converter2/1 -> Data/1
  connections:
  Voltage Sensor3/LConn1 -- V+/RConn1
  Voltage Sensor3/RConn2 -- V-/RConn1
  PS-Simulink Converter2/LConn1 -- Voltage Sensor3/RConn1

== system HalfBridgeCapacitanceModeled/GaN_Bot/Voltage Measure3 ==
  PS-Simulink Converter2 : nesl_utility/PS-Simulink Converter  PhysicalDomain=network_engine_domain  SubClassName=ps_output  LeftPortType=input  RightPortType=output  PseudoPeriodic=off  Frequencies=[]  Unit=1  AffineConversion=off
  Voltage Sensor3 : fl_lib/Electrical/Electrical Sensors/Voltage Sensor
  V+ : PMIOPort  Port=1  Side=Right
  V- : PMIOPort  Port=2  Side=Right
  Data : Outport
  wires:
  PS-Simulink Converter2/1 -> Data/1
  connections:
  PS-Simulink Converter2/LConn1 -- Voltage Sensor3/RConn1
  Voltage Sensor3/RConn2 -- V-/RConn1
  Voltage Sensor3/LConn1 -- V+/RConn1

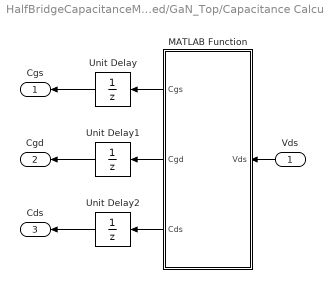
== system HalfBridgeCapacitanceModeled/GaN_Top/Capacitance Calculator ==
  Vds : Inport
  MATLAB Function : MATLAB Function  TreatAsAtomicUnit=on
  Unit Delay : UnitDelay  InitialCondition=258e-12  SampleTime=-1
  Unit Delay1 : UnitDelay  InitialCondition=63e-12  SampleTime=-1
  Unit Delay2 : UnitDelay  InitialCondition=2e-12  SampleTime=-1
  Cgs : Outport
  Cgd : Outport  Port=2
  Cds : Outport  Port=3
  wires:
  Vds/1 -> MATLAB Function/1(Vds)
  MATLAB Function/1(Cgs) -> Unit Delay/1
  MATLAB Function/2(Cgd) -> Unit Delay1/1
  MATLAB Function/3(Cds) -> Unit Delay2/1
  Unit Delay/1 -> Cgs/1
  Unit Delay1/1 -> Cgd/1
  Unit Delay2/1 -> Cds/1

== system HalfBridgeCapacitanceModeled/GaN_Top/Capacitance1 ==
  c : Inport
  Simulink-PS Converter : nesl_utility/Simulink-PS Converter  PhysicalDomain=network_engine_domain  SubClassName=ps_input  LeftPortType=input  RightPortType=output  PseudoPeriodic=off  Frequencies=[]  NoiseDistribution=none  NoiseParameters=[]  Unit=1  AffineConversion=off  InputFiltering=off  SimscapeFilterOrder=1  InputFilterTimeConstant=0.001  UdotUserProvided=1
  Variable Capacitor : elec_lib/Passive Devices/Variable Capacitor  prm=2  Cmin=1e-13 F  r=1e-6 Ohm  v0=0 V  q0=0 c
  C+ : PMIOPort  Port=1  Side=Left
  C- : PMIOPort  Port=2  Side=Right
  wires:
  c/1 -> Simulink-PS Converter/1
  connections:
  Variable Capacitor/LConn1 -- Simulink-PS Converter/RConn1
  Variable Capacitor/LConn2 -- C+/RConn1
  Variable Capacitor/RConn1 -- C-/RConn1

== system HalfBridgeCapacitanceModeled/GaN_Top/Capacitance2 ==
  c : Inport
  Simulink-PS Converter : nesl_utility/Simulink-PS Converter  PhysicalDomain=network_engine_domain  SubClassName=ps_input  LeftPortType=input  RightPortType=output  PseudoPeriodic=off  Frequencies=[]  NoiseDistribution=none  NoiseParameters=[]  Unit=1  AffineConversion=off  InputFiltering=off  SimscapeFilterOrder=1  InputFilterTimeConstant=0.001  UdotUserProvided=1
  Variable Capacitor : elec_lib/Passive Devices/Variable Capacitor  prm=2  Cmin=1e-13 F  r=1e-6 Ohm  v0=0 V  q0=0 c
  C+ : PMIOPort  Port=1  Side=Left
  C- : PMIOPort  Port=2  Side=Right
  wires:
  c/1 -> Simulink-PS Converter/1
  connections:
  Variable Capacitor/RConn1 -- C-/RConn1
  Variable Capacitor/LConn2 -- C+/RConn1
  Variable Capacitor/LConn1 -- Simulink-PS Converter/RConn1

== system HalfBridgeCapacitanceModeled/GaN_Top/Capacitance3 ==
  c : Inport
  Simulink-PS Converter : nesl_utility/Simulink-PS Converter  PhysicalDomain=network_engine_domain  SubClassName=ps_input  LeftPortType=input  RightPortType=output  PseudoPeriodic=off  Frequencies=[]  NoiseDistribution=none  NoiseParameters=[]  Unit=1  AffineConversion=off  InputFiltering=off  SimscapeFilterOrder=1  InputFilterTimeConstant=0.001  UdotUserProvided=1
  Variable Capacitor : elec_lib/Passive Devices/Variable Capacitor  prm=2  Cmin=1e-13 F  r=1e-6 Ohm  v0=0 V  q0=0 c
  C+ : PMIOPort  Port=1  Side=Left
  C- : PMIOPort  Port=2  Side=Right
  wires:
  c/1 -> Simulink-PS Converter/1
  connections:
  Variable Capacitor/RConn1 -- C-/RConn1
  Variable Capacitor/LConn2 -- C+/RConn1
  Variable Capacitor/LConn1 -- Simulink-PS Converter/RConn1
